simulink model "dataStore"  (R2022b)
settings: Solver=VariableStepAuto  StartTime=0.0  StopTime=15  RelTol=1e-3
undefined symbols (not defined in the file): LF
libraries: instrumentseriallib x2
settings Model: Creator=eic20nr  LastModifiedBy=nikilesh
settings ModelReferenceCC: EnableRefExpFcnMdlSchedulingChecks=on

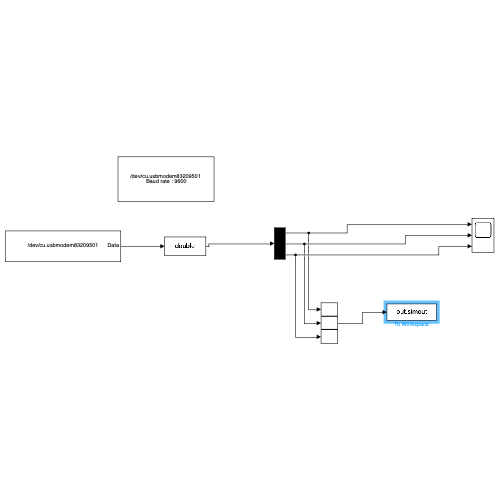
[thumbnail: Simulink's stored preview of the top-level diagram]
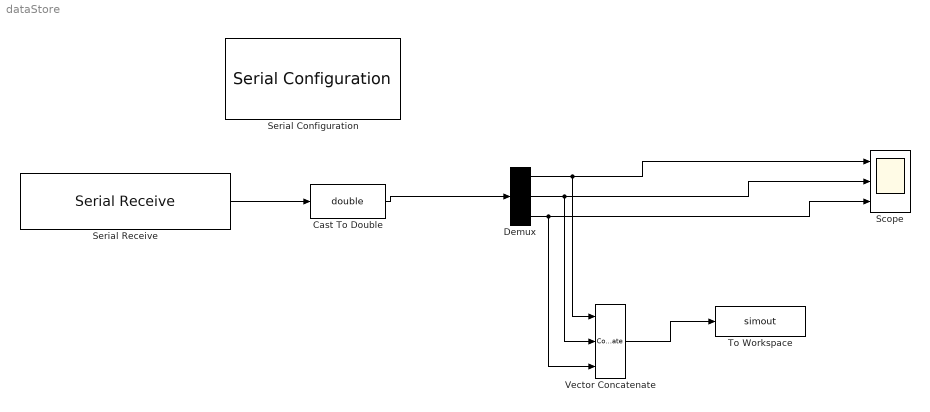
== system dataStore ==
  Cast To Double : DataTypeConversion  OutDataTypeStr=double  SaturateOnIntegerOverflow=off  RndMeth=Floor
  Demux : Demux  Outputs=3
  Scope : Scope  NumInputPorts=3
  Serial Configuration : instrumentseriallib/Serial Configuration  Priority=-200000  PortSel=/dev/cu.usbmodem83209501  Port=/dev/cu.usbmodem83209501  ComPort=/dev/cu.usbmodem83209501  BaudRate=9600  DataBits=8  Parity=none  StopBits=1  ByteOrder=little-endian  FlowControl=none  Timeout=10  SimulateUsing=Interpreted execution  BlockInModel=on  aMode=1
  Serial Receive : instrumentseriallib/Serial Receive  Priority=1  PortSel=/dev/cu.usbmodem83209501  Port=/dev/cu.usbmodem83209501  ComPort=/dev/cu.usbmodem83209501  DataType=single  SaveDataType=uint8  ToggleHeader=on  Header='A'  ToggleTerminator=on  Terminator=LF ('\n')  CustomTerminator=[]  InputFormat=Column major  ToggleDataSize=on  DataSize=[1 3]  EnableBlockingMode=on  ActionDataUnavailable=Output last received value  ActionWhenDataUnavailable=Output last received value  CustomValue=0  SampleTime=0.05  SimulateUsing=Interpreted execution  BlockInModel=on  aMode=1
  To Workspace : ToWorkspace  VariableName=simout  SampleTime=-1
  Vector Concatenate : Concatenate  NumInputs=3
  wires:
  Serial Receive/1 -> Cast To Double/1
  Cast To Double/1 -> Demux/1
  Demux/1 -> Vector Concatenate/1, Scope/1
  Demux/2 -> Vector Concatenate/2, Scope/2
  Demux/3 -> Vector Concatenate/3, Scope/3
  Vector Concatenate/1 -> To Workspace/1
